simulink model "Part6_Vehicle_Behavioral_Planner_using_Stateflow"  (R2021a)
settings: Solver=VariableStepAuto  StartTime=0.0  StopTime=100  RelTol=1e-3
libraries: vrlib x2, simulink x1, mpcadaslib x1
settings Model: Creator=QZHAN112  LastModifiedBy=QZHAN112

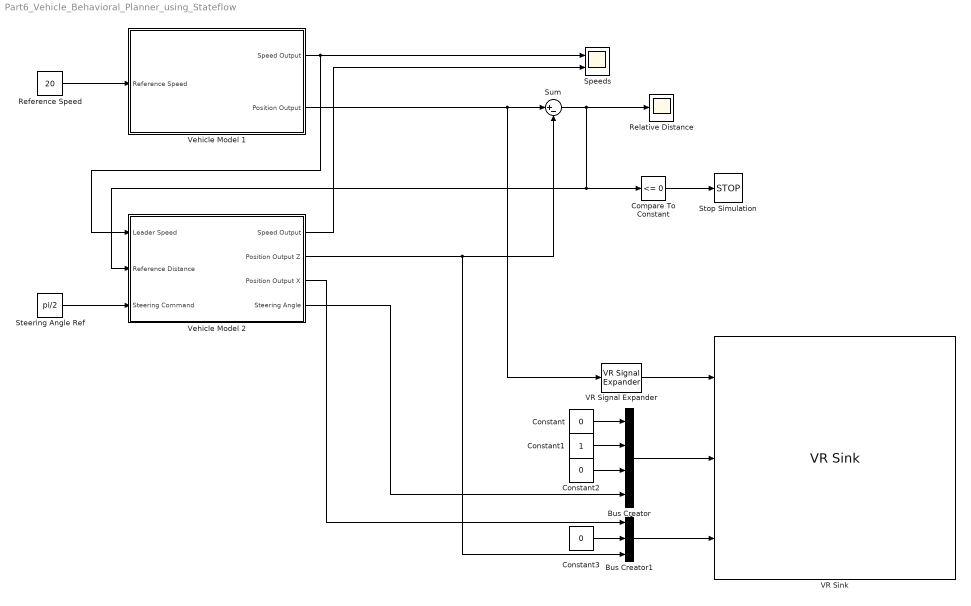
== system Part6_Vehicle_Behavioral_Planner_using_Stateflow ==
  Bus Creator : BusCreator  Inputs=4
  Bus Creator1 : BusCreator  Inputs=3
  Compare To Constant : simulink/Logic and Bit Operations/Compare To Constant  relop=<=  const=0  OutDataTypeStr=boolean
  Constant : Constant  Value=0
  Constant1 : Constant
  Constant2 : Constant  Value=0
  Constant3 : Constant  Value=0
  Reference Speed : Constant  Value=20
  Relative Distance : Scope
  Speeds : Scope  NumInputPorts=2
  Steering Angle Ref : Constant  Value=pi/2
  Stop Simulation : Stop
  Sum : Sum  Inputs=|+-
  VR Signal Expander : vrlib/VR Signal Expander  outwidth=3  outidx=[3]
  VR Sink : vrlib/VR Sink  InstantiateOnLoad=on  SampleTime=0.05  ViewEnable=on  RemoteChange=off  RemoteView=off  FieldsWritten=Car_Red.translation.3.1.1.double#Car_Blue.rotation.4.1.1.double#Car_Blue.translation.3.1.1.double  WorldFileName=PlatoonWorld.WRL  AutoView=off  VideoDimensions=[]  AllowVariableSize=off
  Vehicle Model 1 : Subsystem  mask{Pos=30, Speed=15}
      mask prompts: Pos "Initial Position"; Speed "Initial Speed"
      mask TypeOptions Pos: Initial Position/Value
      mask TypeOptions Speed: Initial Speed/Value
      mask Display: image('model-based autonomous traffic simulation framework\Scratch.jpg');
  Vehicle Model 2 : Subsystem  mask{Pos=0, Speed=30}
      mask prompts: Pos "Initial Position"; Speed "Initial Speed"
      mask TypeOptions Pos: Initial Position Z/Value
      mask TypeOptions Speed: Initial Speed/Value
      mask Display: image('model-based autonomous traffic simulation framework\Car-Design-Drawing-From-Shoulder.jpg');
  wires:
  Vehicle Model 1/2(Position Output) -> Sum/1, VR Signal Expander/1
  Reference Speed/1 -> Vehicle Model 1/1(Reference Speed)
  Vehicle Model 2/1(Speed Output) -> Speeds/2
  Vehicle Model 1/1(Speed Output) -> Speeds/1, Vehicle Model 2/1(Leader Speed)
  Sum/1 -> Relative Distance/1, Compare To Constant/1, Vehicle Model 2/2(Reference Distance)
  Vehicle Model 2/2(Position Output Z) -> Sum/2, Bus Creator1/3
  Compare To Constant/1 -> Stop Simulation/1
  Steering Angle Ref/1 -> Vehicle Model 2/3(Steering Command)
  VR Signal Expander/1 -> VR Sink/1
  Bus Creator1/1 -> VR Sink/3
  Vehicle Model 2/4(Steering Angle) -> Bus Creator/4
  Bus Creator/1 -> VR Sink/2
  Constant/1 -> Bus Creator/1
  Constant1/1 -> Bus Creator/2
  Constant2/1 -> Bus Creator/3
  Constant3/1 -> Bus Creator1/2
  Vehicle Model 2/3(Position Output X) -> Bus Creator1/1

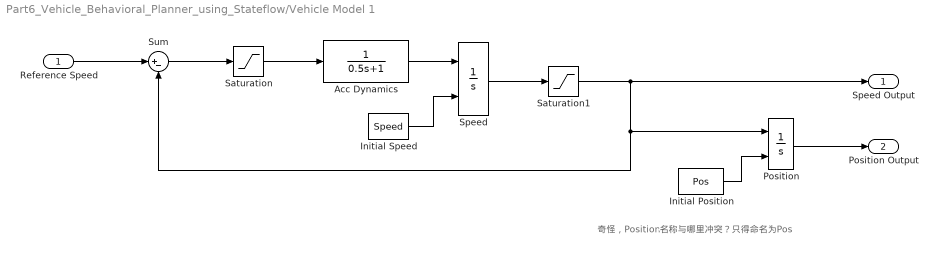
== system Part6_Vehicle_Behavioral_Planner_using_Stateflow/Vehicle Model 1 ==
  note: 奇怪，Position名称与哪里冲突？只得命名为Pos
  Reference Speed : Inport
  Acc Dynamics : TransferFcn  Denominator=[0.5 1]
  Initial Position : Constant  Value=Pos
  Initial Speed : Constant  Value=Speed
  Position : Integrator  InitialConditionSource=external
  Saturation : Saturate  UpperLimit=2  LowerLimit=-3
  Saturation1 : Saturate  UpperLimit=inf  LowerLimit=0
  Speed : Integrator  InitialConditionSource=external
  Sum : Sum  Inputs=|+-
  Speed Output : Outport
  Position Output : Outport  Port=2
  wires:
  Saturation/1 -> Acc Dynamics/1
  Acc Dynamics/1 -> Speed/1
  Speed/1 -> Saturation1/1
  Position/1 -> Position Output/1
  Saturation1/1 -> Speed Output/1, Sum/2, Position/1
  Reference Speed/1 -> Sum/1
  Initial Speed/1 -> Speed/2
  Sum/1 -> Saturation/1
  Initial Position/1 -> Position/2

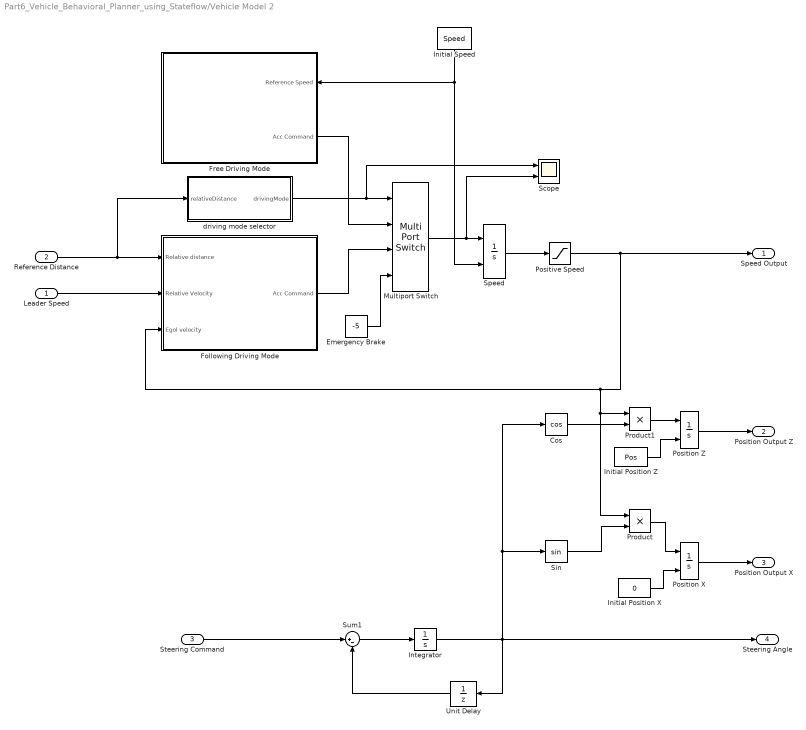
== system Part6_Vehicle_Behavioral_Planner_using_Stateflow/Vehicle Model 2 ==
  Leader Speed : Inport
  Reference Distance : Inport  Port=2
  Steering Command : Inport  Port=3
  Cos : Trigonometry  Operator=cos
  Emergency Brake : Constant  Value=-5
  Following Driving Mode : Subsystem
  Free Driving Mode : Subsystem
      settings: PortSchema="{\"entries\":[{\"content\":{\"sides\":[{\"content\":{\"connectorIds\":[]},\"type\":\"ConnectorPlacement.EquallySpacedRectSide\",\"uuid\":\"610b25c5-b833-48d8-91de-4e4522f1e869\"},{\"content\":{\"connectorIds\":[\"In1\",\"Out1\"],\"side\":\"RIGHT\"},\"type\":\"ConnectorPlacement.EquallySpacedRectSide\",\"uuid\":\"bfbfafdf-9638-4c83-9a6c-a30c0fb24eff\"},{\"content\":{\"connectorIds\":[],\"side\":\"TOP\"},\"type\":\"ConnectorPlacement.EquallySpacedRectSide\",\"uuid\":\"2708cd9c-977e-4237-a5bd-2827f533dc12\"}]},\"type\":\"ConnectorPlacement.EquallySpacedConnector\",\"uuid\":\"23ea83fe-0fb5-46b9-9450-330af3b093f3\"}],\"packageUris\":[\"http://schema.mathworks.com/mf0/Connector/R2020b\"],\"version\":\"1.0\"}"
  Initial Position X : Constant  Value=0
  Initial Position Z : Constant  Value=Pos
  Initial Speed : Constant  Value=Speed
  Integrator : Integrator
  Multiport Switch : MultiPortSwitch
  Position X : Integrator  InitialConditionSource=external
  Position Z : Integrator  InitialConditionSource=external
  Positive Speed : Saturate  UpperLimit=inf  LowerLimit=0
  Product : Product
  Product1 : Product
  Scope : Scope  NumInputPorts=2
  Sin : Trigonometry
  Speed : Integrator  InitialConditionSource=external
  Sum1 : Sum  Inputs=|+-
  Unit Delay : UnitDelay  SampleTime=-1  HasFrameUpgradeWarning=on
  driving mode selector : Stateflow chart  TreatAsAtomicUnit=on
  Speed Output : Outport
  Position Output Z : Outport  Port=2
  Position Output X : Outport  Port=3
  Steering Angle : Outport  Port=4
  wires:
  Speed/1 -> Positive Speed/1
  Position Z/1 -> Position Output Z/1
  Initial Speed/1 -> Speed/2, Free Driving Mode/1(Reference Speed)
  Initial Position Z/1 -> Position Z/2
  Positive Speed/1 -> Speed Output/1, Following Driving Mode/3(Egol velocity), Product/1, Product1/1
  Sum1/1 -> Integrator/1
  Steering Command/1 -> Sum1/1
  Integrator/1 -> Steering Angle/1, Cos/1, Sin/1, Unit Delay/1
  Unit Delay/1 -> Sum1/2
  Sin/1 -> Product/2
  Initial Position X/1 -> Position X/2
  Position X/1 -> Position Output X/1
  Product/1 -> Position X/1
  Cos/1 -> Product1/2
  Product1/1 -> Position Z/1
  Reference Distance/1 -> driving mode selector/1(relativeDistance), Following Driving Mode/1(Relative distance)
  Leader Speed/1 -> Following Driving Mode/2(Relative Velocity)
  Following Driving Mode/1(Acc Command) -> Multiport Switch/3
  Free Driving Mode/1(Acc Command) -> Multiport Switch/2
  Multiport Switch/1 -> Scope/2, Speed/1
  Emergency Brake/1 -> Multiport Switch/4
  driving mode selector/1(drivingMode) -> Scope/1, Multiport Switch/1

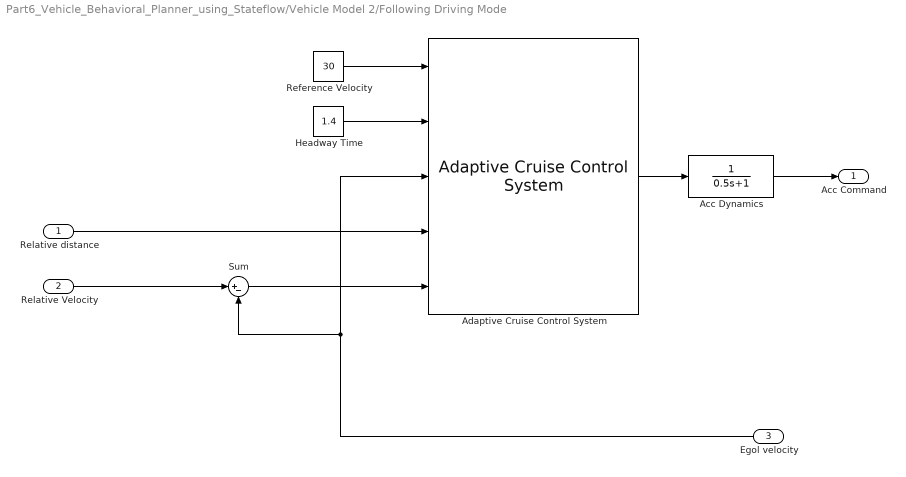
== system Part6_Vehicle_Behavioral_Planner_using_Stateflow/Vehicle Model 2/Following Driving Mode ==
  Relative distance : Inport
  Relative Velocity : Inport  Port=2
  Egol velocity : Inport  Port=3
  Acc Dynamics : TransferFcn  Denominator=[0.5 1]
  Adaptive Cruise Control System : mpcadaslib/Adaptive Cruise Control System  EgoModel=tf(1,[0.5,1,0])  InitialEgoVelocity=30  DefaultSpacing=10  MaxVelocity=50  MinAcceleration=-3  amin_ext=off  MaxAcceleration=2  amax_ext=off  Ts=0.1  PredictionHorizon=300  ControllerBehavior=0.800  suboptimal=off  maxiter=10  datatypeopt=double  optmode=off  trackmode=off
  Headway Time : Constant  Value=1.4
  Reference Velocity : Constant  Value=30
  Sum : Sum  Inputs=|+-
  Acc Command : Outport
  wires:
  Adaptive Cruise Control System/1 -> Acc Dynamics/1
  Sum/1 -> Adaptive Cruise Control System/5
  Reference Velocity/1 -> Adaptive Cruise Control System/1
  Relative distance/1 -> Adaptive Cruise Control System/4
  Egol velocity/1 -> Adaptive Cruise Control System/3, Sum/2
  Relative Velocity/1 -> Sum/1
  Headway Time/1 -> Adaptive Cruise Control System/2
  Acc Dynamics/1 -> Acc Command/1

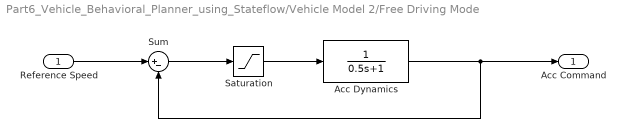
== system Part6_Vehicle_Behavioral_Planner_using_Stateflow/Vehicle Model 2/Free Driving Mode ==
  Reference Speed : Inport
  Acc Dynamics : TransferFcn  Denominator=[0.5 1]
  Saturation : Saturate  UpperLimit=2  LowerLimit=-3
  Sum : Sum  Inputs=|+-
  Acc Command : Outport
  wires:
  Saturation/1 -> Acc Dynamics/1
  Acc Dynamics/1 -> Sum/2, Acc Command/1
  Sum/1 -> Saturation/1
  Reference Speed/1 -> Sum/1

== stateflow chart Part6_Vehicle_Behavioral_Planner_using_Stateflow/Vehicle Model 2/driving mode selector ==
  state FollowingMode
    entry:
    drivingMode = 2;
  state FreeMode
    entry:
    drivingMode = 1;
  state EmergencyBrake
    entry:
    drivingMode = 3;
  (default) -> FreeMode
  FollowingMode -> FreeMode [order 1] : [relativeDistance > 60]
  FreeMode -> FollowingMode [order 1] : [relativeDistance <= 50]
  FreeMode -> EmergencyBrake [order 2] : [relativeDistance <= 25]
  FollowingMode -> EmergencyBrake [order 2] : [relativeDistance <= 25]
  EmergencyBrake -> FollowingMode : [relativeDistance >= 30]
  data: drivingMode output; relativeDistance input
